simulink model "lab1_task_simulink"  (R2016a)
settings: Solver=VariableStepAuto  StartTime=0.0  StopTime=10.0  RelTol=1e-3
settings Model: Creator=Karim  LastModifiedBy=Karim

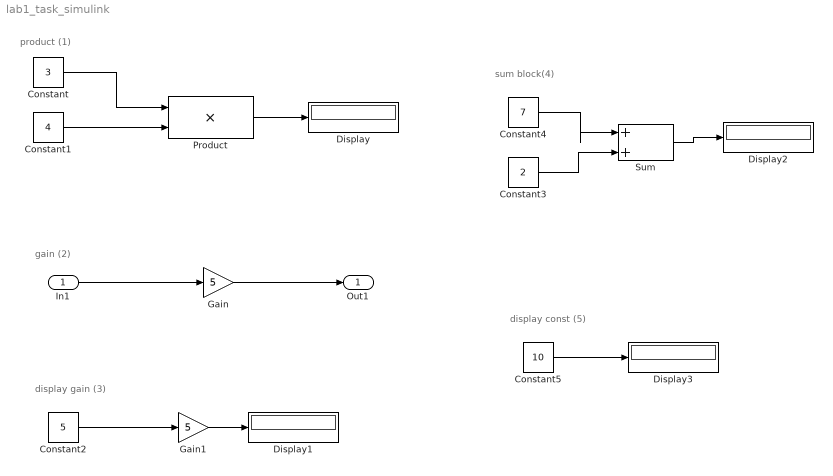
== system lab1_task_simulink ==
  note: display const (5)
  note: sum block(4)
  note: display gain (3)
  note: gain (2)
  note: product (1)
  In1 : Inport
  Constant : Constant  Value=3
  Constant1 : Constant  Value=4
  Constant2 : Constant  Value=5
  Constant3 : Constant  Value=2
  Constant4 : Constant  Value=7
  Constant5 : Constant  Value=10
  Display{,1..3} (4 alike) : Display
  Gain : Gain  Gain=5
  Gain1 : Gain  Gain=5
  Product : Product
  Sum : Sum  Inputs=|++
  Out1 : Outport
  wires:
  Constant/1 -> Product/1
  Constant1/1 -> Product/2
  Product/1 -> Display/1
  In1/1 -> Gain/1
  Gain/1 -> Out1/1
  Constant2/1 -> Gain1/1
  Gain1/1 -> Display1/1
  Constant4/1 -> Sum/1
  Constant3/1 -> Sum/2
  Sum/1 -> Display2/1
  Constant5/1 -> Display3/1
